simulink model "M_INS"  (R2022a)
settings: Solver=ode4  StartTime=0.0  StopTime=0.04  FixedStep=0.01  RelTol=1e-3
PreLoadFcn:
  | listing = dir;
  | if (contains([listing .name], 'INS')) && (contains([listing .name], 'MAP'))
  |     addpath('./INS', './MAP', './DYN');
  |     addpath( genpath('./MAP') );
  | elseif (contains([listing .name], 'M_INS.slx'))
  |     addpath('../INS', '../MAP', '../DYN');
  |     addpath( genpath('../MAP') );
  | else
  | 
  | end
  | 
  | load('BUS_STRUCTURE_INS.mat');
  | load('BUS_STRUCTURE_DYN.mat');
InitFcn:
  | listing = dir;
  | if (contains([listing .name], 'INS')) && (contains([listing .name], 'MAP'))
  |     addpath('./INS', './MAP', './DYN');
  |     addpath( genpath('./MAP') );
  | elseif (contains([listing .name], 'M_INS.slx'))
  |     addpath('../INS', '../MAP', '../DYN');
  |     addpath( genpath('../MAP') );
  | else
  | 
  | end
  | 
  | load('BUS_STRUCTURE_INS.mat');
  | load('BUS_STRUCTURE_DYN.mat');
  | 
  | % Random number seed
  | if ~exist('ranNumSeed', 'var')
  |     ranNumSeed = 2034;
  | end
undefined symbols (not defined in the file or in its folder): f16data
libraries: simulink_extras x13
settings Model: Creator=ASCL  LastModifiedBy=ASCL
settings DataIOCC: SaveOutput=off  SignalLogging=off  DSMLogging=off  SaveTime=off  ReturnWorkspaceOutputs=off
settings OptimizationCC: BlockReduction=off  DefaultParameterBehavior=Inlined  UseDivisionForNetSlopeComputation=on  GainParamInheritBuiltInType=on  UseFloatMulNetSlope=on  ExpressionFolding=off  PassReuseOutputArgsAs=Individual arguments  ZeroExternalMemoryAtStartup=off  ZeroInternalMemoryAtStartup=off  EfficientFloat2IntCast=on  LifeSpan=inf  OptimizeBlockOrder=speed  DifferentSizesBufferReuse=on  EfficientTunableParamExpr=on
settings DebuggingCC: SignalInfNanChecking=warning  ReadBeforeWriteMsg=EnableAllAsError  WriteAfterWriteMsg=EnableAllAsError  WriteAfterReadMsg=EnableAllAsError  IntegerOverflowMsg=error  ParameterTunabilityLossMsg=error  UniqueDataStoreMsg=error  AssertControl=DisableAll  NonBusSignalsTreatedAsBus=error  SFInvalidInputDataAccessInChartInitDiag=error  SFTransitionOutsideNaturalParentDiag=error  SFUnreachableExecutionPathDiag=error  SFUndirectedBroadcastEventsDiag=error  IntegerSaturationMsg=error
settings HardwareCC: ProdBitPerPointer=32  ProdBitPerSizeT=32  ProdBitPerPtrDiffT=32  ProdLargestAtomicInteger=Long  ProdLargestAtomicFloat=Double  ProdEndianess=BigEndian  ProdWordSize=32  ProdLongLongMode=on  ProdHWDeviceType=Freescale->MPC83xx
settings ModelReferenceCC: ModelReferenceNumInstancesAllowed=Single
settings SFSimCC: CompileTimeRecursionLimit=0  EnableRuntimeRecursion=off  MATLABDynamicMemAlloc=off
settings RTWCC: SystemTargetFile=ert.tlc  TemplateMakefile=ert_default_tmf  GenerateReport=on  RTWUseSimCustomCode=on  BuildConfiguration=Faster Runs  IncludeHyperlinkInReport=on  LaunchReport=on  GenerateTraceInfo=on  GenerateTraceReport=on  GenerateTraceReportSl=on  GenerateTraceReportSf=on  GenerateTraceReportEml=on
settings CodeAppCC: ForceParamTrailComments=on  IgnoreCustomStorageClasses=off  OperatorAnnotations=on  SimulinkDataObjDesc=on  SFDataObjDesc=on  MATLABFcnDesc=on  InsertBlockDesc=on  StateflowObjectComments=on  MATLABSourceComments=on  EnableCustomComments=on  InlinedPrmAccess=Macros  ReqsInCode=on
settings ERTTargetCC: TargetLangStandard=C99 (ISO)  UtilityFuncGeneration=Shared location  GenerateSampleERTMain=on  IncludeMdlTerminateFcn=off  CombineSignalStateStructs=on  SupportAbsoluteTime=off  SupportNonFinite=off  SupportVariableSizeSignals=on  ParenthesesLevel=Standards  CastingMode=Standards  GenerateSharedConstants=off  InlinedParameterPlacement=NonHierarchical  ERTCustomFileTemplate=example_file_process.tlc  RateTransitionBlockCode=Function  PreserveIfCondition=on  ConvertIfToSwitch=off  EnableSignedLeftShifts=off  EnableSignedRightShifts=off

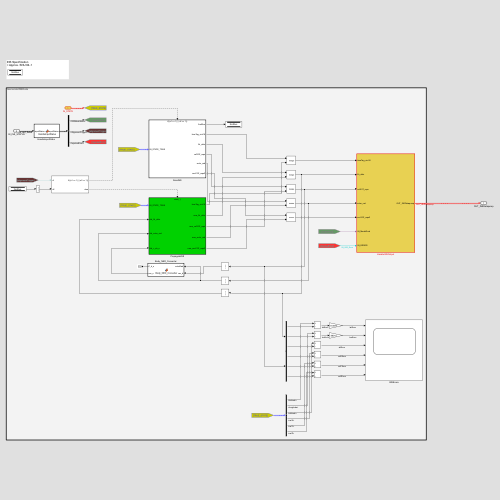
[thumbnail: Simulink's stored preview of the top-level diagram]
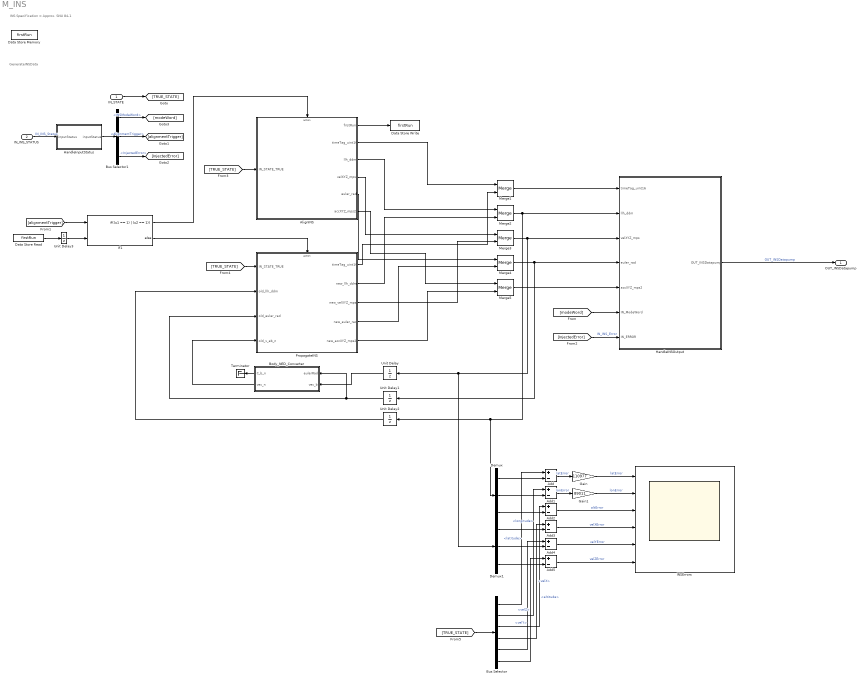
== system M_INS ==
  note: GenerateINSData
  note: INS Specification
      | = Approx. SNU 84-1
  IN_STATE : Inport  OutDataTypeStr=Bus: BUS_DYN_STATE  Interpolate=off  BusOutputAsStruct=on
  IN_INS_STATUS : Inport  Port=2  OutDataTypeStr=Bus: BUS_SENSOR_INS_INPUTSTATUS  Interpolate=off  BusOutputAsStruct=on
  Add{,1..5} (6 alike) : Sum  Inputs=+-
  AlignINS : Subsystem  TreatAsAtomicUnit=on
      settings: RTWSystemCode=Nonreusable function  RTWFcnNameOpts=Use subsystem name
  Body_NED_Converter : MATLAB Function  TreatAsAtomicUnit=on
  Bus Selector : BusSelector  OutputSignals=latitude,longitude,altitude,velX,velY,velZ
  Bus Selector1 : BusSelector  OutputSignals=INSModeWord,AlignmentTrigger,InjectedError
  Data Store Memory : DataStoreMemory  DataStoreName=firstRun  ReadBeforeWriteMsg=warning  WriteAfterWriteMsg=warning  WriteAfterReadMsg=warning  InitialValue=logical(1)  VectorParams1D=off  ShowAdditionalParam=off  OutDataTypeStr=boolean
      settings: LockScale=on
  Data Store Read : DataStoreRead  DataStoreName=firstRun  IndexOptions=Index vector (dialog)  Indices=1  OutputSizes=1
  Data Store Write : DataStoreWrite  DataStoreName=firstRun  IndexOptions=Index vector (dialog)  Indices=1  OutputSizes=1
  Demux : Demux  Outputs=3
  Demux1 : Demux  Outputs=3
  Gain : Gain  Gain=110977
  Gain1 : Gain  Gain=89011
  HandleINSOutput : Subsystem  TreatAsAtomicUnit=on
      settings: RTWSystemCode=Nonreusable function  RTWFcnNameOpts=Use subsystem name
  HandleInputStatus : MATLAB Function  TreatAsAtomicUnit=on
  INSErrors : Scope  NumInputPorts=6
  If1 : If  NumInputs=2  IfExpression=(u1 == 1) | (u2 == 1)
  Merge{1..5} (5 alike) : Merge
  PropagateINS : Subsystem  TreatAsAtomicUnit=on
      settings: RTWSystemCode=Nonreusable function  RTWFcnNameOpts=Use subsystem name
  Terminator : Terminator
  Unit Delay : UnitDelay  SampleTime=-1  HasFrameUpgradeWarning=on
  Unit Delay1 : UnitDelay  SampleTime=-1  HasFrameUpgradeWarning=on
  Unit Delay2 : UnitDelay  SampleTime=-1  HasFrameUpgradeWarning=on
  Unit Delay3 : UnitDelay  InitialCondition=logical(1)  SampleTime=-1  HasFrameUpgradeWarning=on
  OUT_INSDatapump : Outport  OutDataTypeStr=Bus: BUS_SENSOR_INS_DP  VectorParamsAs1DForOutWhenUnconnected=off  BusOutputAsStruct=on
  wires:
  IN_INS_STATUS/1 -> HandleInputStatus/1("inputStatus ")  "IN_INS_Status"
  IN_STATE/1 -> [TRUE_STATE]
  Bus Selector1/2 -> [alignmentTrigger]  "<AlignmentTrigger>"
  Bus Selector1/3 -> [InjectedError]  "<InjectedError>"
  HandleInputStatus/1(inputStatus) -> Bus Selector1/1
  Bus Selector1/1 -> [modeWord]  "<INSModeWord>"
  [modeWord] -> HandleINSOutput/6(IN_ModeWord)
  HandleINSOutput/1(OUT_INSDatapump) -> OUT_INSDatapump/1  "OUT_INSDatapump"
  Merge1/1 -> HandleINSOutput/1(timeTag_uint16)
  Add/1 -> Gain/1  "latError"
  Bus Selector/6 -> Add5/1  "<velZ>"
  Demux1/3 -> Add5/2
  Bus Selector/2 -> Add1/1  "<longitude>"
  Demux/1 -> Add/2
  Bus Selector/3 -> Add2/1  "<altitude>"
  [InjectedError] -> HandleINSOutput/7(IN_ERROR)  "IN_INS_Error"
  Demux/3 -> Add2/2
  Add1/1 -> Gain1/1  "lonError"
  Gain1/1 -> INSErrors/2  "lonError"
  Add3/1 -> INSErrors/4  "velXError"
  PropagateINS/3(new_velXYZ_mps) -> Merge3/2
  AlignINS/2(timeTag_uint16) -> Merge1/1
  PropagateINS/4(new_euler_rad) -> Merge4/2
  Demux/2 -> Add1/2
  Data Store Read/1 -> Unit Delay3/1
  Add5/1 -> INSErrors/6  "velZError"
  [alignmentTrigger] -> If1/1
  AlignINS/5(euler_rad) -> Merge4/1
  If1/2 -> PropagateINS/Action
  Add2/1 -> INSErrors/3  "altError"
  AlignINS/1(firstRun) -> Data Store Write/1
  If1/1 -> AlignINS/Action
  AlignINS/4(velXYZ_mps) -> Merge3/1
  AlignINS/3(llh_ddm) -> Merge2/1
  Demux1/1 -> Add3/2
  Bus Selector/1 -> Add/1  "<latitude>"
  Unit Delay/1 -> Body_NED_Converter/2(vec_b)
  PropagateINS/1(timeTag_uint16) -> Merge1/2
  Body_NED_Converter/1(C_b_n) -> Terminator/1
  Demux1/2 -> Add4/2
  Unit Delay2/1 -> PropagateINS/2(old_llh_ddm)
  Merge3/1 -> Demux1/1, Unit Delay/1, HandleINSOutput/3(velXYZ_mps)
  Gain/1 -> INSErrors/1  "latError"
  AlignINS/6(accXYZ_mps2) -> Merge5/1
  Bus Selector/5 -> Add4/1  "<velY>"
  Merge2/1 -> HandleINSOutput/2(llh_ddm), Demux/1, Unit Delay2/1
  Body_NED_Converter/2(vec_n) -> PropagateINS/4(old_v_eb_n)
  Unit Delay3/1 -> If1/2
  Add4/1 -> INSErrors/5  "velYError"
  PropagateINS/5(new_accXYZ_mps2) -> Merge5/2
  Bus Selector/4 -> Add3/1  "<velX>"
  PropagateINS/2(new_llh_ddm) -> Merge2/2
  Merge5/1 -> HandleINSOutput/5(accXYZ_mps2)
  Merge4/1 -> Unit Delay1/1, HandleINSOutput/4(euler_rad)
  Unit Delay1/1 -> PropagateINS/3(old_euler_rad), Body_NED_Converter/1(eulerRad)
  [TRUE_STATE] -> AlignINS/1(IN_STATE_TRUE)
  [TRUE_STATE] -> PropagateINS/1(IN_STATE_TRUE)
  [TRUE_STATE] -> Bus Selector/1

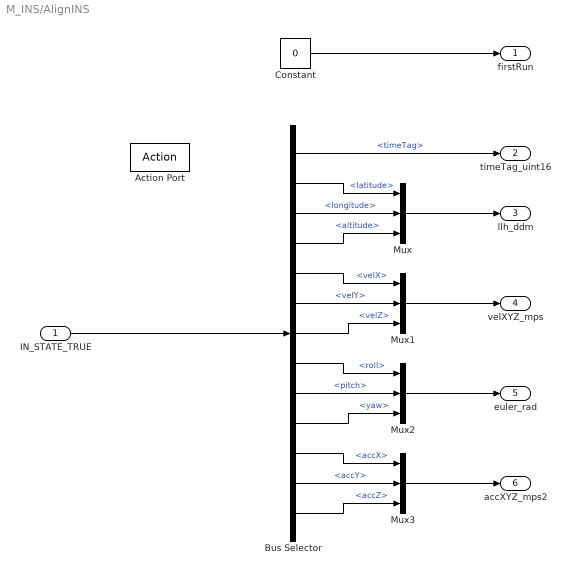
== system M_INS/AlignINS ==
  IN_STATE_TRUE : Inport  OutDataTypeStr=Bus: BUS_DYN_STATE
  Action Port : ActionPort  ActionPortLabel=if((u1 == 1) | (u2 == 1))
  Bus Selector : BusSelector  OutputSignals=timeTag,latitude,longitude,altitude,velX,velY,velZ,roll,pitch,yaw,accX,accY,accZ
  Constant : Constant  Value=0  OutDataTypeStr=boolean
  Mux{,1..3} (4 alike) : Mux  Inputs=3
  firstRun : Outport
  timeTag_uint16 : Outport  Port=2
  llh_ddm : Outport  Port=3
  velXYZ_mps : Outport  Port=4
  euler_rad : Outport  Port=5
  accXYZ_mps2 : Outport  Port=6
  wires:
  IN_STATE_TRUE/1 -> Bus Selector/1
  Bus Selector/1 -> timeTag_uint16/1  "<timeTag>"
  Bus Selector/3 -> Mux/2  "<longitude>"
  Bus Selector/2 -> Mux/1  "<latitude>"
  Bus Selector/4 -> Mux/3  "<altitude>"
  Bus Selector/13 -> Mux3/3  "<accZ>"
  Bus Selector/11 -> Mux3/1  "<accX>"
  Bus Selector/12 -> Mux3/2  "<accY>"
  Bus Selector/9 -> Mux2/2  "<pitch>"
  Bus Selector/10 -> Mux2/3  "<yaw>"
  Bus Selector/8 -> Mux2/1  "<roll>"
  Bus Selector/7 -> Mux1/3  "<velZ>"
  Bus Selector/6 -> Mux1/2  "<velY>"
  Bus Selector/5 -> Mux1/1  "<velX>"
  Mux3/1 -> accXYZ_mps2/1
  Mux2/1 -> euler_rad/1
  Mux1/1 -> velXYZ_mps/1
  Mux/1 -> llh_ddm/1
  Constant/1 -> firstRun/1

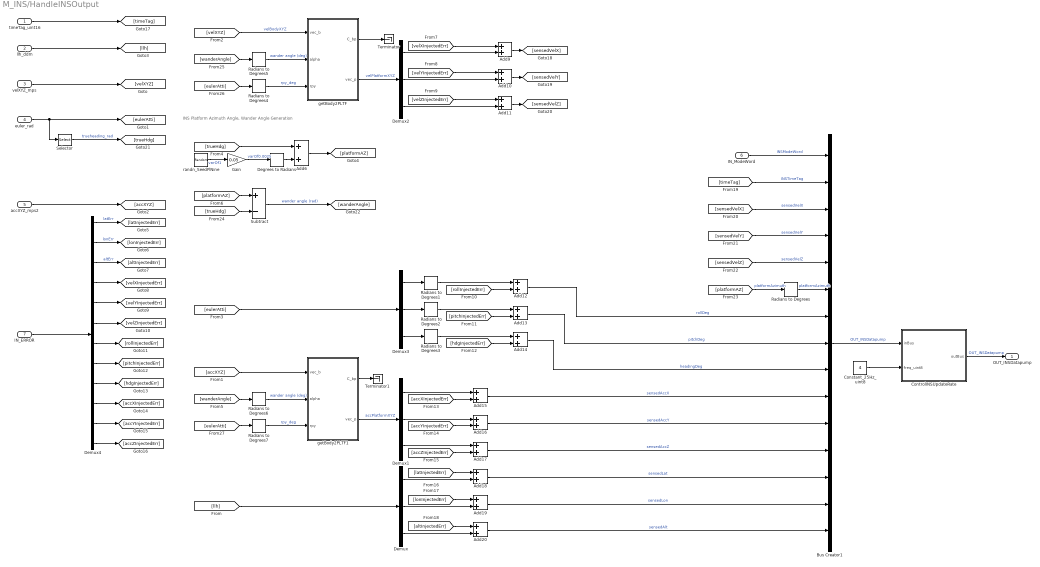
== system M_INS/HandleINSOutput ==
  note: INS Platform Azimuth Angle, Wander Angle Generation
  timeTag_uint16 : Inport  OutDataTypeStr=uint16
  llh_ddm : Inport  Port=2
  velXYZ_mps : Inport  Port=3
  euler_rad : Inport  Port=4
  accXYZ_mps2 : Inport  Port=5
  IN_ModeWord : Inport  Port=6
  IN_ERROR : Inport  Port=7
  Add{6,9..20} (13 alike) : Sum
  Bus Creator1 : BusCreator  Inputs=15  OutDataTypeStr=Bus: BUS_SENSOR_INS_DP  NonVirtualBus=on
      settings: InheritFromInputs=off
  Constant_25Hz_uint8 : Constant  Value=4  OutDataTypeStr=uint8
  ControlINSUpdateRate : MATLAB Function  TreatAsAtomicUnit=on  SystemSampleTime=0.01
  Degrees to Radians : simulink_extras/Transformations/Degrees to Radians
  Demux{,1..3} (4 alike) : Demux  Outputs=3
  Demux4 : Demux  Outputs=12
  Gain : Gain  Gain=0.05
  Radians to Degrees{,1..7} (8 alike) : simulink_extras/Transformations/Radians to Degrees
  Selector : Selector  InputPortWidth=3  IndexOptions=Index vector (dialog)  Indices=[3]  OutputSizes=1
  Subtract : Sum  Inputs=+-
  Terminator : Terminator
  Terminator1 : Terminator
  getBody2PLTF : MATLAB Function  TreatAsAtomicUnit=on
  getBody2PLTF1 : MATLAB Function  TreatAsAtomicUnit=on
  randn_SeedPlNine : RandomNumber  Seed=(ranNumSeed+9)  SampleTime=0.01
  OUT_INSDatapump : Outport  OutDataTypeStr=Bus: BUS_SENSOR_INS_DP
  wires:
  IN_ModeWord/1 -> Bus Creator1/1  "INSModeWord"
  timeTag_uint16/1 -> [timeTag]
  Demux2/1 -> Add9/2
  Demux2/3 -> Add11/2
  Demux1/1 -> Add15/1
  Demux1/2 -> Add16/1
  Demux1/3 -> Add17/1
  Demux/1 -> Add18/2
  Demux/2 -> Add19/2
  Demux/3 -> Add20/2
  Demux3/1 -> Radians to Degrees1/1
  Demux3/2 -> Radians to Degrees2/1
  Demux3/3 -> Radians to Degrees3/1
  velXYZ_mps/1 -> [velXYZ]
  accXYZ_mps2/1 -> [accXYZ]
  llh_ddm/1 -> [llh]
  [llh] -> Demux/1
  [eulerAtti] -> Demux3/1
  Add6/1 -> [platformAZ]
  Demux2/2 -> Add10/2
  [accXYZ] -> getBody2PLTF1/1(vec_b)
  getBody2PLTF1/2(vec_p) -> Demux1/1  "accPlatformXYZ"
  [velXYZ] -> getBody2PLTF/1(vec_b)  "velBodyXYZ"
  IN_ERROR/1 -> Demux4/1
  Demux4/1 -> [latInjectedErr]  "latErr"
  Demux4/2 -> [lonInjectedErr]  "lonErr"
  Demux4/3 -> [altInjectedErr]  "altErr"
  Demux4/4 -> [velXInjectedErr]
  Demux4/5 -> [velYInjectedErr]
  Demux4/6 -> [velZInjectedErr]
  Demux4/7 -> [rollInjectedErr]
  Demux4/8 -> [pitchInjectedErr]
  Demux4/9 -> [hdgInjectedErr]
  Demux4/12 -> [accZInjectedErr]
  Demux4/11 -> [accYInjectedErr]
  Demux4/10 -> [accXInjectedErr]
  Add9/1 -> [sensedVelX]
  [velXInjectedErr] -> Add9/1
  Add10/1 -> [sensedVelY]
  [velYInjectedErr] -> Add10/1
  Add11/1 -> [sensedVelZ]
  [velZInjectedErr] -> Add11/1
  [pitchInjectedErr] -> Add13/2
  [rollInjectedErr] -> Add12/2
  [hdgInjectedErr] -> Add14/2
  Add15/1 -> Bus Creator1/10  "sensedAccX"
  Add16/1 -> Bus Creator1/11  "sensedAccY"
  Add17/1 -> Bus Creator1/12  "sensedAccZ"
  [accXInjectedErr] -> Add15/2
  [accYInjectedErr] -> Add16/2
  [accZInjectedErr] -> Add17/2
  [latInjectedErr] -> Add18/1
  [lonInjectedErr] -> Add19/1
  [altInjectedErr] -> Add20/1
  Bus Creator1/1 -> ControlINSUpdateRate/1(inBus)  "OUT_INSDatapump"
  [timeTag] -> Bus Creator1/2  "INSTimeTag"
  [sensedVelX] -> Bus Creator1/3  "sensedVelX"
  [sensedVelY] -> Bus Creator1/4  "sensedVelY"
  [sensedVelZ] -> Bus Creator1/5  "sensedVelZ"
  [platformAZ] -> Radians to Degrees/1  "platformAzimuth"
  Add18/1 -> Bus Creator1/13  "sensedLat"
  Add19/1 -> Bus Creator1/14  "sensedLon"
  Add20/1 -> Bus Creator1/15  "sensedAlt"
  Radians to Degrees/1 -> Bus Creator1/6  "platformAzimuth"
  Add12/1 -> Bus Creator1/7  "rollDeg"
  Add13/1 -> Bus Creator1/8  "pitchDeg"
  Add14/1 -> Bus Creator1/9  "headingDeg"
  Radians to Degrees3/1 -> Add14/1
  Radians to Degrees1/1 -> Add12/1
  Radians to Degrees2/1 -> Add13/1
  Selector/1 -> [trueHdg]  "trueheading_rad"
  randn_SeedPlNine/1 -> Gain/1  "varOf1"
  getBody2PLTF/2(vec_p) -> Demux2/1  "velPlatformXYZ"
  euler_rad/1 -> Selector/1, [eulerAtti]
  getBody2PLTF/1(C_bp) -> Terminator/1
  Subtract/1 -> [wanderAngle]  "wander angle (rad)"
  [platformAZ] -> Subtract/1
  [trueHdg] -> Add6/1
  [trueHdg] -> Subtract/2
  [wanderAngle] -> Radians to Degrees5/1
  Radians to Degrees5/1 -> getBody2PLTF/2(alpha)  "wander angle (deg)"
  getBody2PLTF1/1(C_bp) -> Terminator1/1
  Radians to Degrees6/1 -> getBody2PLTF1/2(alpha)  "wander angle (deg)"
  [wanderAngle] -> Radians to Degrees6/1
  [eulerAtti] -> Radians to Degrees4/1
  Radians to Degrees4/1 -> getBody2PLTF/3(rpy)  "rpy_deg"
  [eulerAtti] -> Radians to Degrees7/1
  Radians to Degrees7/1 -> getBody2PLTF1/3(rpy)  "rpy_deg"
  Gain/1 -> Degrees to Radians/1  "varOf0.0025"
  Degrees to Radians/1 -> Add6/2
  Constant_25Hz_uint8/1 -> ControlINSUpdateRate/2(freq_uint8)
  ControlINSUpdateRate/1(outBus) -> OUT_INSDatapump/1  "OUT_INSDatapump"

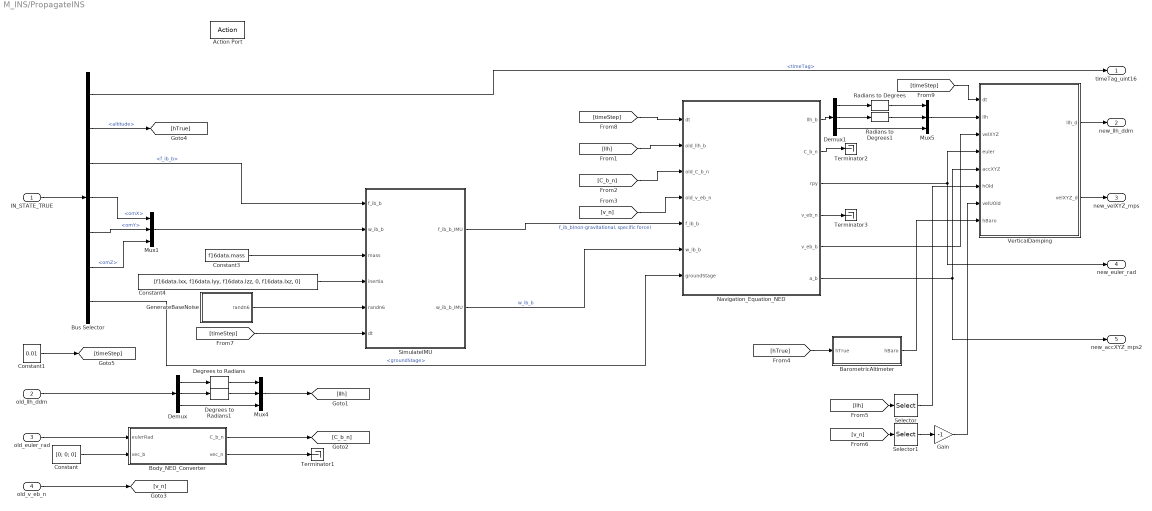
== system M_INS/PropagateINS ==
  IN_STATE_TRUE : Inport  OutDataTypeStr=Bus: BUS_DYN_STATE
  old_llh_ddm : Inport  Port=2
  old_euler_rad : Inport  Port=3
  old_v_eb_n : Inport  Port=4
  Action Port : ActionPort  ActionPortLabel=else
  BarometricAltimeter : Subsystem
  Body_NED_Converter : MATLAB Function  TreatAsAtomicUnit=on
  Bus Selector : BusSelector  OutputSignals=timeTag,altitude,f_ib_b,omX,omY,omZ,groundStage
  Constant : Constant  Value=[0; 0; 0]
  Constant1 : Constant  Value=0.01  OutDataTypeStr=double
  Constant3 : Constant  Value=f16data.mass
  Constant4 : Constant  Value=[f16data.Ixx, f16data.Iyy, f16data.Izz, 0, f16data.Ixz, 0]
  Degrees to Radians : simulink_extras/Transformations/Degrees to Radians
  Degrees to Radians1 : simulink_extras/Transformations/Degrees to Radians
  Demux : Demux  Outputs=3
  Demux1 : Demux  Outputs=3
  Gain : Gain  Gain=-1
  GenerateBaseNoise : Subsystem
  Mux1 : Mux  Inputs=3
  Mux4 : Mux  Inputs=3
  Mux5 : Mux  Inputs=3
  Navigation_Equation_NED : MATLAB Function  TreatAsAtomicUnit=on
      settings: RTWSystemCode=Nonreusable function  RTWFcnNameOpts=Use subsystem name
  Radians to Degrees : simulink_extras/Transformations/Radians to Degrees
  Radians to Degrees1 : simulink_extras/Transformations/Radians to Degrees
  Selector : Selector  InputPortWidth=3  IndexOptions=Index vector (dialog)  Indices=3  OutputSizes=1
  Selector1 : Selector  InputPortWidth=3  IndexOptions=Index vector (dialog)  Indices=3  OutputSizes=1
  SimulateIMU : MATLAB Function  TreatAsAtomicUnit=on
      settings: RTWSystemCode=Nonreusable function  RTWFcnNameOpts=Use subsystem name
  Terminator1 : Terminator
  Terminator2 : Terminator
  Terminator3 : Terminator
  VerticalDamping : MATLAB Function  TreatAsAtomicUnit=on
  timeTag_uint16 : Outport
  new_llh_ddm : Outport  Port=2
  new_velXYZ_mps : Outport  Port=3
  new_euler_rad : Outport  Port=4
  new_accXYZ_mps2 : Outport  Port=5
  wires:
  Bus Selector/4 -> Mux1/1  "<omX>"
  IN_STATE_TRUE/1 -> Bus Selector/1
  Bus Selector/6 -> Mux1/3  "<omZ>"
  Bus Selector/2 -> [hTrue]  "<altitude>"
  [timeStep] -> Navigation_Equation_NED/1(dt)
  Bus Selector/5 -> Mux1/2  "<omY>"
  old_llh_ddm/1 -> Demux/1
  old_euler_rad/1 -> Body_NED_Converter/1(eulerRad)
  old_v_eb_n/1 -> [v_n]
  [v_n] -> Navigation_Equation_NED/4(old_v_eb_n)
  [llh] -> Navigation_Equation_NED/2(old_llh_b)
  Body_NED_Converter/1(C_b_n) -> [C_b_n]
  Body_NED_Converter/2(vec_n) -> Terminator1/1
  Bus Selector/1 -> timeTag_uint16/1  "<timeTag>"
  Degrees to Radians/1 -> Mux4/1
  Demux/1 -> Degrees to Radians/1
  Demux/2 -> Degrees to Radians1/1
  Degrees to Radians1/1 -> Mux4/2
  Demux/3 -> Mux4/3
  Mux4/1 -> [llh]
  Radians to Degrees1/1 -> Mux5/2
  Demux1/1 -> Radians to Degrees/1
  Demux1/2 -> Radians to Degrees1/1
  Demux1/3 -> Mux5/3
  Radians to Degrees/1 -> Mux5/1
  Navigation_Equation_NED/2(C_b_n) -> Terminator2/1
  Navigation_Equation_NED/3(rpy) -> VerticalDamping/4(euler), new_euler_rad/1
  Navigation_Equation_NED/5(v_eb_b) -> VerticalDamping/3(velXYZ)
  Navigation_Equation_NED/6(a_b) -> VerticalDamping/5(accXYZ), new_accXYZ_mps2/1
  Navigation_Equation_NED/4(v_eb_n) -> Terminator3/1
  Navigation_Equation_NED/1(llh_b) -> Demux1/1
  Mux5/1 -> VerticalDamping/2(llh)
  Constant/1 -> Body_NED_Converter/2(vec_b)
  SimulateIMU/2(w_ib_b_IMU) -> Navigation_Equation_NED/6(w_ib_b)  "w_ib_b"
  VerticalDamping/1(llh_d) -> new_llh_ddm/1
  VerticalDamping/2(velXYZ_d) -> new_velXYZ_mps/1
  BarometricAltimeter/1(hBaro) -> VerticalDamping/8(hBaro)
  [hTrue] -> BarometricAltimeter/1(hTrue)
  [llh] -> Selector/1
  Selector/1 -> VerticalDamping/6(hOld)
  [v_n] -> Selector1/1
  Selector1/1 -> Gain/1
  Gain/1 -> VerticalDamping/7(velUOld)
  GenerateBaseNoise/1(randn6) -> SimulateIMU/5(randn6)
  Constant1/1 -> [timeStep]
  [timeStep] -> SimulateIMU/6(dt)
  [timeStep] -> VerticalDamping/1(dt)
  SimulateIMU/1(f_ib_b_IMU) -> Navigation_Equation_NED/5(f_ib_b)  "f_ib_b(non-gravitational, specific force)"
  Bus Selector/3 -> SimulateIMU/1(f_ib_b)  "<f_ib_b>"
  Constant3/1 -> SimulateIMU/3(mass)
  Constant4/1 -> SimulateIMU/4(inertia)
  Mux1/1 -> SimulateIMU/2(w_ib_b)
  [C_b_n] -> Navigation_Equation_NED/3(old_C_b_n)
  Bus Selector/7 -> Navigation_Equation_NED/7(groundStage)  "<groundStage>"

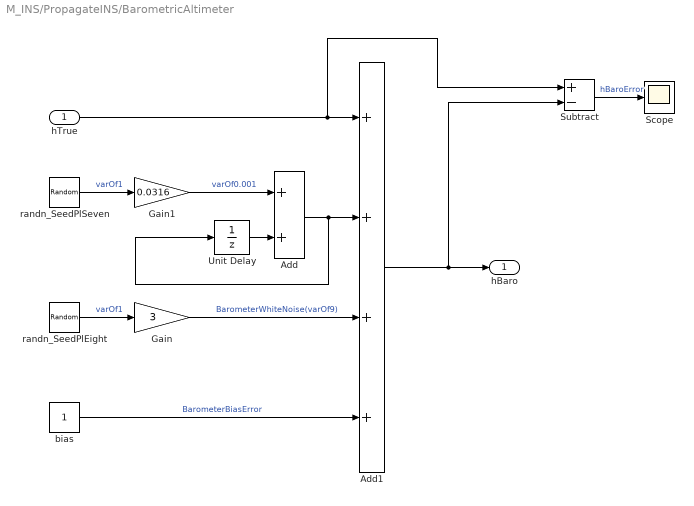
== system M_INS/PropagateINS/BarometricAltimeter ==
  hTrue : Inport
  Add : Sum
  Add1 : Sum  Inputs=++++
  Gain : Gain  Gain=3
  Gain1 : Gain  Gain=0.0316
  Scope : Scope
  Subtract : Sum  Inputs=+-
  Unit Delay : UnitDelay  SampleTime=-1  HasFrameUpgradeWarning=on
  bias : Constant
  randn_SeedPlEight : RandomNumber  Seed=(ranNumSeed+8)  SampleTime=0.01
  randn_SeedPlSeven : RandomNumber  Seed=(ranNumSeed+7)  SampleTime=0.01
  hBaro : Outport
  wires:
  hTrue/1 -> Subtract/1, Add1/1
  Add1/1 -> Subtract/2, hBaro/1
  Gain1/1 -> Add/1  "varOf0.001"
  Gain/1 -> Add1/3  "BarometerWhiteNoise(varOf9)"
  Add/1 -> Unit Delay/1, Add1/2
  Unit Delay/1 -> Add/2
  bias/1 -> Add1/4  "BarometerBiasError"
  randn_SeedPlSeven/1 -> Gain1/1  "varOf1"
  randn_SeedPlEight/1 -> Gain/1  "varOf1"
  Subtract/1 -> Scope/1  "hBaroError"

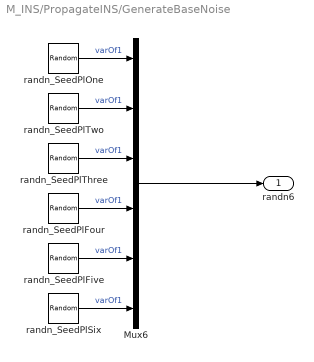
== system M_INS/PropagateINS/GenerateBaseNoise ==
  Mux6 : Mux  Inputs=6
  randn_SeedPlFive : RandomNumber  Seed=(ranNumSeed+5)  SampleTime=0.01
  randn_SeedPlFour : RandomNumber  Seed=(ranNumSeed+4)  SampleTime=0.01
  randn_SeedPlOne : RandomNumber  Seed=(ranNumSeed+1)  SampleTime=0.01
  randn_SeedPlSix : RandomNumber  Seed=(ranNumSeed+6)  SampleTime=0.01
  randn_SeedPlThree : RandomNumber  Seed=(ranNumSeed+3)  SampleTime=0.01
  randn_SeedPlTwo : RandomNumber  Seed=(ranNumSeed+2)  SampleTime=0.01
  randn6 : Outport
  wires:
  randn_SeedPlOne/1 -> Mux6/1  "varOf1"
  randn_SeedPlSix/1 -> Mux6/6  "varOf1"
  randn_SeedPlFour/1 -> Mux6/4  "varOf1"
  randn_SeedPlTwo/1 -> Mux6/2  "varOf1"
  randn_SeedPlFive/1 -> Mux6/5  "varOf1"
  randn_SeedPlThree/1 -> Mux6/3  "varOf1"
  Mux6/1 -> randn6/1

== matlab function M_INS/PropagateINS/VerticalDamping ==
  data: dt input; llh input; velXYZ input; euler input; accXYZ input; hOld input; velUOld input; hBaro input; llh_d output; velXYZ_d output
function [llh_d, velXYZ_d] = VerticalDamping(dt, llh, velXYZ, euler, accXYZ, hOld, velUOld, hBaro)

% Initialize
llh_d = zeros(3,1);
velXYZ_d = zeros(3,1);
velNED = zeros(3,1);
accNED = zeros(3,1);

% Transform
velNED = ConvertBody2NED(euler, velXYZ);
accNED = ConvertBody2NED(euler, accXYZ);

% Rearrange
velU = - velNED(3);
h = llh(3);
accU = - accNED(3);

% Time constant
tau = 25;
% Schuler frequency
w_s = 0.00124;

% Gains
K1 = 3/tau;
K2 = 3/tau^2 + 2*w_s^2;
K3 = 1/tau^3;

%
velUDot = accU + 2*w_s^2*h - K2*(h-hBaro) - K3*(h-hBaro)*dt;
velU = velUOld + velUDot*dt;
hDot = velU - K1*(h-hBaro);
h = hOld + hDot*dt;

% Output
llh_d = llh;
llh_d(3) = h;

velNED(3) = - velU;
% accNED(3) = aD;

velXYZ_d = ConvertNED2Body(euler, velNED);

% accXYZ_d = ConvertNED2Body(accNED);

end


function vec_n = ConvertBody2NED(eulerRad, vec_b)

vec_n = zeros(3,1);
C_b_n  = zeros(3,3);

% Body to NED
cRol = cos(eulerRad(1));
sRol = sin(eulerRad(1));
cPit = cos(eulerRad(2));
sPit = sin(eulerRad(2));
cYaw = cos(eulerRad(3));
sYaw = sin(eulerRad(3));

C_b_n   = [ cPit*cYaw, sRol*sPit*cYaw-cRol*sYaw, cRol*sPit*cYaw+sRol*sYaw;...
            cPit*sYaw, sRol*sPit*sYaw+cRol*cYaw, cRol*sPit*sYaw-sRol*cYaw;...
                -sPit,                sRol*cPit,                cRol*cPit];

vec_n  = C_b_n * vec_b;

end

function vec_b = ConvertNED2Body(eulerRad, vec_n)

vec_b = zeros(3,1);
C_n_b  = zeros(3,3);

% Body to NED
cRol = cos(eulerRad(1));
sRol = sin(eulerRad(1));
cPit = cos(eulerRad(2));
sPit = sin(eulerRad(2));
cYaw = cos(eulerRad(3));
sYaw = sin(eulerRad(3));

C_n_b   = [              cPit*cYaw,                cPit*sYaw,     -sPit;...
          sRol*sPit*cYaw-cRol*sYaw, sRol*sPit*sYaw+cRol*cYaw, sRol*cPit;...
          cRol*sPit*cYaw+sRol*sYaw, cRol*sPit*sYaw-sRol*cYaw, cRol*cPit];

vec_b  = C_n_b * vec_n;

end

== matlab function M_INS/HandleInputStatus ==
  data: inputStatus input Bus: BUS_SENSOR_INS_INPUTSTATUS; inputStatus output
function inputStatus = HandleInputStatus(inputStatus)

if(inputStatus.InputActivated)
    
else
    inputStatus.INSModeWord = uint16(0b0000000000000000);
    inputStatus.AlignmentTrigger = false;
end

== matlab function M_INS/HandleINSOutput/getBody2PLTF1 ==
  data: vec_b input; C_bp output; alpha input; rpy input; vec_p output
function [C_bp, vec_p] = getBody2PLTF(vec_b, alpha, rpy)
%getBody2PLTF Convert a vector in body axis to INS Platform axis
%
% Inputs
%   vec_b   : a vector in body axis (3x1)
%   alpha   : wander angle "platform azimuth - true heading" (deg)
%   rpy     : roll, pitch, yaw(true heading) angles (deg)
%
% Outputs
%   C_bp    : computed tranformation matrix from body to INS Platform axis 
%   vec_p   : converted vec_b in INS platform axis

% Initialize
C_bp = zeros(3,3);
vec_p = zeros(3,1);

% Arrange
cRol = cosd(rpy(1));
sRol = sind(rpy(1));
cPit = cosd(rpy(2));
sPit = sind(rpy(2));
cYaw = cosd(rpy(3));
sYaw = sind(rpy(3));

% Transformation matrix form INS Platform axis to local NED navigation
% frame
C_np = [ cosd(alpha), -sind(alpha),  0; ...
        -sind(alpha), -cosd(alpha),  0; ...
                   0,            0, -1];

% Transformation matrix from local NED to body
C_bn   = [ cPit*cYaw, sRol*sPit*cYaw-cRol*sYaw, cRol*sPit*cYaw+sRol*sYaw;...
           cPit*sYaw, sRol*sPit*sYaw+cRol*cYaw, cRol*sPit*sYaw-sRol*cYaw;...
               -sPit,                sRol*cPit,                cRol*cPit];

C_bp = C_np * C_bn;

% Convert a given vector to platform axis
vec_p = C_bp * vec_b;

end

== matlab function M_INS/PropagateINS/Body_NED_Converter ==
  data: eulerRad input; C_b_n output; vec_n output; vec_b input
function [C_b_n, vec_n] = Body_NED_Converter(eulerRad, vec_b)

vec_n = zeros(3,1);
C_b_n = zeros(3,3);

% Body to NED
cRol = cos(eulerRad(1));
sRol = sin(eulerRad(1));
cPit = cos(eulerRad(2));
sPit = sin(eulerRad(2));
cYaw = cos(eulerRad(3));
sYaw = sin(eulerRad(3));

C_n_b   = [              cPit*cYaw,                cPit*sYaw,     -sPit;...
          sRol*sPit*cYaw-cRol*sYaw, sRol*sPit*sYaw+cRol*cYaw, sRol*cPit;...
          cRol*sPit*cYaw+sRol*sYaw, cRol*sPit*sYaw-sRol*cYaw, cRol*cPit];

C_b_n = C_n_b';

      
vec_n  = C_n_b * vec_b;


end

== matlab function M_INS/PropagateINS/SimulateIMU ==
  data: f_ib_b input; w_ib_b input; mass input; inertia input; randn6 input; dt input; f_ib_b_IMU output; w_ib_b_IMU output
function [f_ib_b_IMU, w_ib_b_IMU] = SimulateIMU(f_ib_b, w_ib_b, mass, inertia, randn6, dt)
%SIMULATEIMU
% == INPUT
% accXYZ
% omXYZ
% == OUTPUT
% f_ib_b_IMU
% w_ib_b_IMU

%% Constans & Noise characteristics
muG                 = 9.8E-6;               % [m/s^2]
accl_noise_root_PSD = 20 * muG;             % [m/s^1.5]
gyro_noise_root_PSD = 0.002 * (pi/180) / 60;% [rad/s^0.5]
tor_i               = dt;                   % [sec]

persistent old_w_ib_b
if isempty(old_w_ib_b)
    old_w_ib_b = zeros(3,1);
end

w_ib_b_IMU = zeros(3,1);
f_ib_b_IMU = zeros(3,1);

% Ib      = [inertia(1), -inertia(4), -inertia(5);...
%           -inertia(4),  inertia(2), -inertia(6);...
%           -inertia(5), -inertia(6),  inertia(3)];
% 
% w_dot_ib_b = zeros(3,1);
% w_dot_ib_b = Ib\(M_ib_b - cross(old_w_ib_b, Ib*old_w_ib_b));
% w_ib_b     = old_w_ib_b + dt * w_dot_ib_b;
% 
% % Store w_ib_b before noise added
% old_w_ib_b = w_ib_b;
% 
% f_ib_b = F_ib_b / mass;

% Accelerometer biases (micro-g, converted to m/s^2; body axes)
% b_a = [80; -110; 70] * muG;
% Assume Horizontal acceleration biases are unobservable during initial
% alignment.
% b_a = [25; -30; -5] * muG;
b_a = [25; -30; -5] * muG;

% Gyro biases (deg/hour, converted to rad/sec; body axes)
% b_g     = [-0.09; 0.013; -0.08] * (pi/180) / 3600;
% Assume all gyro axis measurements are observable
b_g     = [-0.0004; 0.0005; -0.0005] * (pi/180) / 3600;

% Accelerometer scale factor and cross coupling errors (ppm, converted to
% unitless; body axes)
% M_a     = [500, -300, 200;
%           -150, -600, 250;
%           -250,  100, 450] * 1E-6;
M_a     = [100, -120,  80;
           -60, -120, 100;
          -100,  40,   90] * 1E-6;

% Gyro scale factor and cross coupling errors (ppm, converted to unitless;
% body axes)  ~10^(-5) for RLGs.
% M_g     = [8,   80, -95;
%            0,   -9,  65;
%            0,    0,  -5] * 1E-6;
M_g     = [2,   20, -25;
           0,   -3,  15;
           0,    0,  -1] * 1E-6;

% Gyro g-dependent biases (deg/hour/g, converted to rad-sec/m; body axes)
% RLG, FOG exhibit no g-dependenet biases
% G_g     = [0.9, -1.1, -0.6;
%           -0.5,  1.9, -1.6;
%            0.3,  1.1, -1.3] * (pi/180) / (3600 * 9.8);          
G_g     = zeros(3,3);

% randn6 = zeros(6,1);
%% Generate Noise
accl_noise = randn6(1:3, 1) * accl_noise_root_PSD / sqrt(tor_i);
gyro_noise = randn6(4:6, 1) * gyro_noise_root_PSD / sqrt(tor_i);

% current measurements
f_ib_b_IMU   = b_a + (eye(3) + M_a) * f_ib_b + accl_noise;
w_ib_b_IMU   = b_g + (eye(3) + M_g) * w_ib_b + G_g * f_ib_b + gyro_noise;


end

== matlab function M_INS/Body_NED_Converter ==
  data: eulerRad input; C_b_n output; vec_n output; vec_b input
function [C_b_n, vec_n] = Body_NED_Converter(eulerRad, vec_b)

vec_n = zeros(3,1);
C_b_n  = zeros(3,3);

% Body to NED
cRol = cos(eulerRad(1));
sRol = sin(eulerRad(1));
cPit = cos(eulerRad(2));
sPit = sin(eulerRad(2));
cYaw = cos(eulerRad(3));
sYaw = sin(eulerRad(3));

C_n_b   = [              cPit*cYaw,                cPit*sYaw,     -sPit;...
          sRol*sPit*cYaw-cRol*sYaw, sRol*sPit*sYaw+cRol*cYaw, sRol*cPit;...
          cRol*sPit*cYaw+sRol*sYaw, cRol*sPit*sYaw-sRol*cYaw, cRol*cPit];

C_b_n = C_n_b';

      
vec_n  = C_b_n * vec_b;


end

== matlab function M_INS/HandleINSOutput/getBody2PLTF ==
  data: vec_b input; C_bp output; alpha input; rpy input; vec_p output
function [C_bp, vec_p] = getBody2PLTF(vec_b, alpha, rpy)
%getBody2PLTF Convert a vector in body axis to INS Platform axis
%
% Inputs
%   vec_b   : a vector in body axis (3x1)
%   alpha   : wander angle "platform azimuth - true heading" (deg)
%   rpy     : roll, pitch, yaw(true heading) angles (deg)
%
% Outputs
%   C_bp    : computed tranformation matrix from body to INS Platform axis 
%   vec_p   : converted vec_b in INS platform axis

% Initialize
C_bp = zeros(3,3);
vec_p = zeros(3,1);

% Arrange
cRol = cosd(rpy(1));
sRol = sind(rpy(1));
cPit = cosd(rpy(2));
sPit = sind(rpy(2));
cYaw = cosd(rpy(3));
sYaw = sind(rpy(3));

% Transformation matrix form INS Platform axis to local NED navigation
% frame
C_np = [ cosd(alpha), -sind(alpha),  0; ...
        -sind(alpha), -cosd(alpha),  0; ...
                   0,            0, -1];

% Transformation matrix from local NED to body
C_bn   = [ cPit*cYaw, sRol*sPit*cYaw-cRol*sYaw, cRol*sPit*cYaw+sRol*sYaw;...
           cPit*sYaw, sRol*sPit*sYaw+cRol*cYaw, cRol*sPit*sYaw-sRol*cYaw;...
               -sPit,                sRol*cPit,                cRol*cPit];

C_bp = C_np * C_bn;

% Convert a given vector to platform axis
vec_p = C_bp * vec_b;

end

== matlab function M_INS/PropagateINS/Navigation_Equation_NED ==
  data: dt input; llh_b output; old_llh_b input; old_C_b_n input; old_v_eb_n input; f_ib_b input; w_ib_b input; C_b_n output; rpy output; v_eb_n output; v_eb_b output; a_b output; groundStage input
function [llh_b, C_b_n, rpy, v_eb_n, v_eb_b, a_b]   = Navigation_Equation_NED(dt, old_llh_b, old_C_b_n, old_v_eb_n, f_ib_b, w_ib_b, groundStage)
% Reference:    Groves, Paul D. "Principles of GNSS, inertial, and 
%               multisensor integrated navigation systems, [Book review]."
%               IEEE Aerospace and Electronic Systems Magazine 30.2 (2015): 26-27.
%
% INPUTS:
%   dt          time interval between updates [s]
%   old_llh_b   previous latitude, longitude, height [rad, rad, m]
%   old_C_b_n   previous body-to-NED coordinate transformation matrix
%   old_v_eb_n  previous velocity of body frame w.r.t. ECEF frame,
%               resolved along north, east, and down [m/s]
%   f_ib_b      (non-gravitational) force of body frame w.r.t.
%               ECEF frame, resolved along body-frame axes, averaged over
%               time interval [m/s^2]s]
%   w_ib_b      measured body angular rate w.r.t. ECI frame,
%               resolved about body axes [rad/s]
%   inertia     [kg m^2]
%
% OUTPUTS: 
%   llh_b       latitude, longitude, height [rad, rad, m]
%   C_b_n       body-to-NED coordinate transformation matrix
%   v_eb_n      velocity of body frame w.r.t. ECEF frame,
%               resolved along north, east, and down [m/s]
%   a_b         body acceleration [m/s^2]
%   rpy         attitude (roll, pitch, yaw) [rad]
%   v_eb_b      body velocity [m/s]

%% [0] Initialize Outputs
persistent old_w_ib_b
if isempty(old_w_ib_b)
    old_w_ib_b = zeros(3,1);
end

llh_b   = zeros(3,1);
C_b_n   = zeros(3,3);
rpy     = zeros(3,1);
v_eb_n  = zeros(3,1);
v_eb_b  = zeros(3,1);
a_b     = zeros(3,1);

if groundStage == uint8(9)
    llh_b = old_llh_b;
    C_b_n = old_C_b_n;
    return;
end

%% [1] Define Constant Parameters
w_ie    = 7.2921159E-5;     % Earth rotation rate [rad/s]
R_0     = 6378137;          % WGS84 Equatorial radius [m]
R_P     = 6356752.31425;    %WGS84 Polar radius [m]
e       = 0.0818191908425;  % WGS84 eccentricity
f       = 1 / 298.257223563;%WGS84 flattening
mu      = 3.986004418E14;   %WGS84 Earth gravitational constant [m^3 s^-2]

TOL     = eps(0.5);

% Ib      = [inertia(1), -inertia(4), -inertia(5);...
%           -inertia(4),  inertia(2), -inertia(6);...
%           -inertia(5), -inertia(6),  inertia(3)];
%                           % Moment of inertia [kg m^2]

%% [2] ATTITUDE UPDATE

% Calculate w_ib_b: angular rate of body frame w.r.t. ECI frame,
%           resolved about body axes, averaged over time interval [rad/s]
% w_dot_ib_b  = Ib\(M_ib_b - cross(old_w_ib_b, Ib*old_w_ib_b));
% w_ib_b      = old_w_ib_b + 0.5 * dt * (w_dot_ib_b + old_w_dot_ib_b); 

% lumpedS     = [         1,        0;      -sin(euler(2));...
%                         0, cos(euler(
% eulerRate   = 

% First, Calculate attitude increment, magnitude, and skew-symmetric matrix
% alpha_ib_b  = (w_ib_b + old_w_ib_b) * 0.5 * dt;
alpha_ib_b = w_ib_b * dt;
if abs(alpha_ib_b' * alpha_ib_b - 0) < TOL % (alpha_ib_b' * alpha_ib_b == 0)
    mag_alpha   = 0.0;
else
    mag_alpha   = sqrt(alpha_ib_b' * alpha_ib_b);
end

Alpha_ib_b  = [             0, -alpha_ib_b(3),  alpha_ib_b(2); ...
                alpha_ib_b(3),              0, -alpha_ib_b(1); ...
               -alpha_ib_b(2),  alpha_ib_b(1),             0];

w_ie_n      = w_ie * [cos(old_llh_b(1)); 0; -sin(old_llh_b(1))];

% From (5.44), determine the angular rate of the NED frame
% w.r.t the ECEF frame, resolved about NED
% old_N_E     = R_0 * (1-e^2) / sqrt( 1 - (e * sin(old_llh_b(1)))^2 );
% old_M_E     = R_0 / ( 1 - (e * sin(old_llh_b(1)))^2 )^1.5;
old_N_E     = R_0 * (1-e^2) / sqrt( 1 - (e * sin(old_llh_b(1)))^2 );
old_M_E_norm1 = 1 - (e * sin(old_llh_b(1)))^2;
if (old_M_E_norm1 > 0.000001)
    old_M_E_norm2 = sqrt(old_M_E_norm1);
    old_M_E_norm3 = old_M_E_norm1 * old_M_E_norm2;
    old_M_E = R_0 / old_M_E_norm3;
else
    old_M_E_norm2 = 0.0;
    old_M_E_norm3 = 0.0;
    old_M_E = R_0 / 0.97;
end

old_w_en_n = [old_v_eb_n(2) / (old_N_E + old_llh_b(3));...
             -old_v_eb_n(1) / (old_M_E + old_llh_b(3));...
             -old_v_eb_n(2) * tan(old_llh_b(1)) / (old_N_E + old_llh_b(3))];


%% [3] SPECIFIC FORCE FRAME TRANSFORMATION
% Calculate ave_C_b_e: the average body-to-ECEF-frame transformation matrix
%           over the update interval using (5.84) and (5.85)
temp_w_enie_n   = old_w_en_n + w_ie_n;
skew_w_enie_n   = [               0,-temp_w_enie_n(3), temp_w_enie_n(2);...
                   temp_w_enie_n(3),                0,-temp_w_enie_n(1);...
                  -temp_w_enie_n(2), temp_w_enie_n(1),                0];

if (mag_alpha > 1.E-8)
    ave_C_b_n = old_C_b_n * (eye(3) + (1 - cos(mag_alpha)) / mag_alpha^2 ...
        * Alpha_ib_b + (1 - sin(mag_alpha) / mag_alpha) / mag_alpha^2 ...
        * Alpha_ib_b * Alpha_ib_b) ...
        - 0.5 * skew_w_enie_n * old_C_b_n;
else
     ave_C_b_n = old_C_b_n ...
        - 0.5 * skew_w_enie_n * old_C_b_n;
end %if mag_alpha     

% Transform specific force to ECEF-frame resolving axes using (5.86)
f_ib_n = ave_C_b_n * f_ib_b;

%% [4] UPDATE VELOCITY
% Calculate acceleration due to gravity resolved about NED
grav_n = zeros(3,1);

% Calculate surface gravity using the Somigliana model, (2.134)
sinsqL = sin(old_llh_b(1))^2;
g_0 = 9.7803253359 * (1 + 0.001931853 * sinsqL) / sqrt(1 - e^2 * sinsqL);

% Calculate north gravity using (2.140)
grav_n(1) = -8.08E-9 * old_llh_b(3) * sin(2 * old_llh_b(1));

% East gravity is zero
grav_n(2) = 0.0;

% Calculate down gravity using (2.139)
grav_n(3) = g_0 ...
    * (1 - (2 / R_0) * (1 + f * (1 - 2 * sinsqL) + (w_ie^2 * R_0^2 * R_P / mu)) ...
    * old_llh_b(3) + (3 * old_llh_b(3)^2 / R_0^2));

% Calculate Skew-symmetric matrix for Coriolis and transport-rate term
w_CnT   = old_w_en_n + 2 * w_ie_n;
skew_w_CnT  = [       0, -w_CnT(3),  w_CnT(2); ...
               w_CnT(3),         0, -w_CnT(1); ...
              -w_CnT(2),  w_CnT(1),         0];

% From (5.54),
v_eb_n = old_v_eb_n ...
    + dt * f_ib_n ...
    + dt * grav_n ...
    - dt * skew_w_CnT * old_v_eb_n;

%% [5] UPDATE CURVILINEAR POSITION
% Update height using (5.56)
llh_b(3)    = old_llh_b(3) ...
    - dt/2 * (old_v_eb_n(3) + v_eb_n(3));

% Update latitude using (5.56)
llh_b(1)    = old_llh_b(1) ...
    + dt/2 * old_v_eb_n(1) / (old_M_E + old_llh_b(3)) ...
    + dt/2 * v_eb_n(1) / (old_M_E + llh_b(3));

% Calculate meridian and transverse radii of curvature
N_E         = R_0 * (1-e^2) / sqrt( 1 - (e * sin(llh_b(1)))^2 );
% M_E         = R_0 / ( 1 - (e * sin(llh_b(1)))^2 )^1.5;
M_E_norm1 = 1 - (e * sin(llh_b(1)))^2;
if (M_E_norm1 > 0.000001)
    M_E_norm2 = sqrt(M_E_norm1);
    M_E_norm3 = M_E_norm1 * M_E_norm2;
    M_E = R_0 / M_E_norm3;
else
    M_E_norm2 = 0.0;
    M_E_norm3 = 0.0;
    M_E = R_0 / 0.97;
end

% Update longitude using (5.56)
llh_b(2)    = old_llh_b(2) ...
    + dt/2 * old_v_eb_n(2) / ((old_N_E + old_llh_b(3)) * cos(old_llh_b(1))) ...
    + dt/2 * v_eb_n(2) / ((N_E + llh_b(3)) * cos(llh_b(1)));

%% [6] UPDATE ATTITUDE
% From (5.44), determine the angular rate of the NED frame
% w.r.t the ECEF frame, resolved about NED frame
w_en_n  = [v_eb_n(2) / (N_E + llh_b(3));...
          -v_eb_n(1) / (M_E + llh_b(3));...
          -v_eb_n(2) * tan(llh_b(1)) / (N_E + llh_b(3))];

% Obtain coordinate transformation matrix from the new attitude w.r.t. an
% inertial frame to the old using Rodrigues' formula, (5.73)
if mag_alpha>1.E-8
    C_new_old = eye(3) + sin(mag_alpha) / mag_alpha * Alpha_ib_b +...
        (1 - cos(mag_alpha)) / mag_alpha^2 * Alpha_ib_b * Alpha_ib_b;
else
    C_new_old = eye(3) + Alpha_ib_b;
end %if mag_alpha

% Update attitude using (5.77)
ave_w_ie_n  = w_ie_n + 0.5 * w_en_n + 0.5 * old_w_en_n;
skew_w_ie_n = [            0, -ave_w_ie_n(3),  ave_w_ie_n(2); ...
               ave_w_ie_n(3),              0, -ave_w_ie_n(1); ...
              -ave_w_ie_n(2),  ave_w_ie_n(1),              0];

C_b_n   = (eye(3) - skew_w_ie_n * dt) * old_C_b_n * C_new_old;

% Orthonormalize DCM
C_b_n   = quat2rotm(quatnormalize(rotm2quat(C_b_n)));
 
%% [7] CALCULATE EULER ANGLES
C_n_b = C_b_n';

% ERRORPOINT!!!
C23 = C_n_b(2,3);
C33 = C_n_b(3,3);

rpy(1,1) = atan2(C23, C33);  % roll
if isnan(rpy(1,1))
    rpy(1,1) = 0.0;
end
rpy(2,1) = - asin(C_n_b(1,3));        % pitch
rpy(3,1) = atan2(C_n_b(1,2),C_n_b (1,1));  % yaw
if isnan(rpy(3,1))
    rpy(3,1) = 0.0;
end

%% [8] CALCULATE BODY VELOCITY
v_eb_b  = C_n_b * v_eb_n;
a_b = f_ib_b + C_n_b * (grav_n - skew_w_CnT * old_v_eb_n);

old_w_ib_b = w_ib_b;
end

== matlab function M_INS/HandleINSOutput/ControlINSUpdateRate ==
  data: inBus input Bus: BUS_SENSOR_INS_DP; freq_uint8 input uint8; outBus output Bus: BUS_SENSOR_INS_DP
function outBus = ControlINSUpdateRate(inBus, freq_uint8)
%ControlINSUpdateRate INS 데이터 갱신주기 제어
% Input
% - inBus       Datatype: BUS_SENSOR_INS_DP
% - freq_uint8  1 = update data at every simulation step
%               4 = update data at every 4 simulation steps
%               Accepts  (8bit unsigned integer=uint8) only
% Output
% - outBus      Datatype: BUS_SENSOR_INS_DP
persistent tempBus cnt

assert (isa(freq_uint8, 'uint8'))

if isempty(cnt)
    cnt = uint8(0);
end
if isempty(tempBus)
    tempBus = inBus;
end

if mod(cnt, freq_uint8) == uint8(0)
    tempBus = inBus;
    cnt = uint8(1);
else
    cnt = cnt + uint8(1);
end

outBus = tempBus;

end
